simulink model "SimulacaoMassaPonto"  (R2021a)
settings: Solver=VariableStepAuto  StartTime=0.0  StopTime=TVoo  MaxStep=Step  RelTol=1e-3
values from neighbouring files (symbols this model uses):
  g = 9.81    [TesteSimulacaoMP.m]
  Gamma0 = deg2rad(85)    [TesteSimulacaoMP.m]
  Mvazio = 32.3    [TesteSimulacaoMP.m]
  Sref = 0.0196    [TesteSimulacaoMP.m]
  Tq = VProp(end, 1)    [TesteSimulacaoMP.m]
  V0 = 24    [TesteSimulacaoMP.m]
  VCD = [ 0.0 0.3757 ... (first row only)    [TesteSimulacaoMP.m]
  VMass = load('mass.txt')    [TesteSimulacaoMP.m]
  VProp = load('Prop.txt')    [TesteSimulacaoMP.m]
  X0 = deg2rad(45)    [TesteSimulacaoMP.m]
  XEast0 = 0    [TesteSimulacaoMP.m]
  XNorth0 = 0    [TesteSimulacaoMP.m]
  XUp0 = 0    [TesteSimulacaoMP.m]
libraries: simulink x2, simulink_extras x2, aerolibptmass x1, aerolibatmos2 x1
settings Model: Creator=gabriel  LastModifiedBy=gabriel

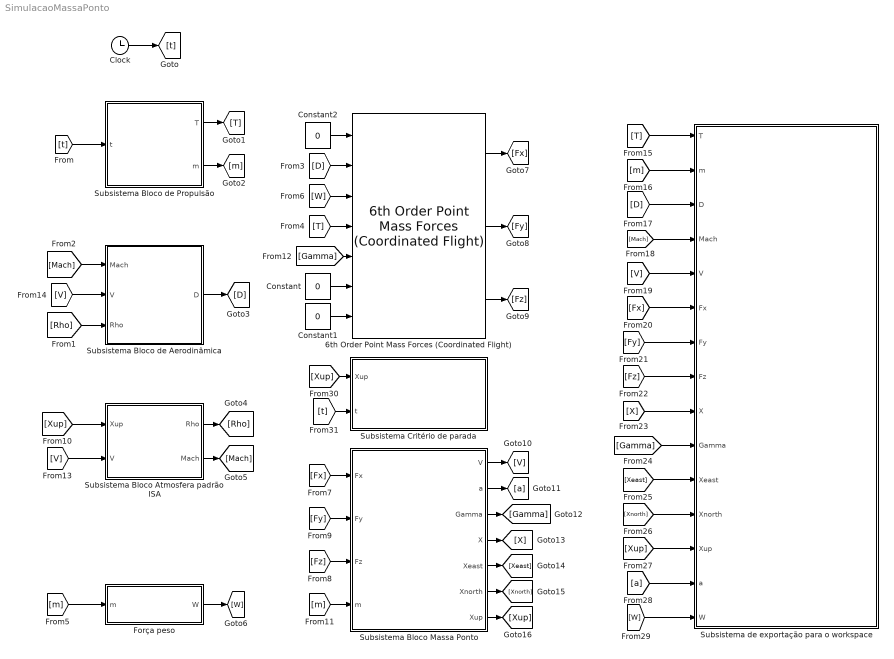
== system SimulacaoMassaPonto ==
  6th Order Point Mass Forces (Coordinated Flight) : aerolibptmass/6th Order Point Mass Forces (Coordinated Flight)
      settings: SourceProductBaseCode=AE
  Clock : Clock
  Constant : Constant  Value=0
  Constant1 : Constant  Value=0
  Constant2 : Constant  Value=0
  Força peso : Subsystem
  Subsistema Bloco Atmosfera padrão ISA : Subsystem
  Subsistema Bloco Massa Ponto : Subsystem
  Subsistema Bloco de Aerodinâmica : Subsystem
  Subsistema Bloco de Propulsão : Subsystem
  Subsistema Critério de parada : Subsystem
  Subsistema de exportação para o workspace : Subsystem
  wires:
  Clock/1 -> [t]
  [t] -> Subsistema Bloco de Propulsão/1(t)
  Subsistema Bloco de Propulsão/1(T) -> [T]
  Subsistema Bloco de Propulsão/2(m) -> [m]
  Subsistema Bloco de Aerodinâmica/1(D) -> [D]
  Subsistema Bloco Atmosfera padrão ISA/1(Rho) -> [Rho]
  [Rho] -> Subsistema Bloco de Aerodinâmica/3(Rho)
  Subsistema Bloco Atmosfera padrão ISA/2(Mach) -> [Mach]
  [Mach] -> Subsistema Bloco de Aerodinâmica/1(Mach)
  [D] -> 6th Order Point Mass Forces (Coordinated Flight)/2
  [T] -> 6th Order Point Mass Forces (Coordinated Flight)/4
  [m] -> Força peso/1(m)
  Força peso/1(W) -> [W]
  [W] -> 6th Order Point Mass Forces (Coordinated Flight)/3
  Constant2/1 -> 6th Order Point Mass Forces (Coordinated Flight)/1
  6th Order Point Mass Forces (Coordinated Flight)/3 -> [Fz]
  6th Order Point Mass Forces (Coordinated Flight)/2 -> [Fy]
  6th Order Point Mass Forces (Coordinated Flight)/1 -> [Fx]
  [Fx] -> Subsistema Bloco Massa Ponto/1(Fx)
  [Fz] -> Subsistema Bloco Massa Ponto/3(Fz)
  [Fy] -> Subsistema Bloco Massa Ponto/2(Fy)
  [m] -> Subsistema Bloco Massa Ponto/4(m)
  Subsistema Bloco Massa Ponto/1(V) -> [V]
  Subsistema Bloco Massa Ponto/2(a) -> [a]
  Subsistema Bloco Massa Ponto/3(Gamma) -> [Gamma]
  [Gamma] -> 6th Order Point Mass Forces (Coordinated Flight)/5
  Constant/1 -> 6th Order Point Mass Forces (Coordinated Flight)/6
  Constant1/1 -> 6th Order Point Mass Forces (Coordinated Flight)/7
  Subsistema Bloco Massa Ponto/4(X) -> [X]
  Subsistema Bloco Massa Ponto/5(Xeast) -> [Xeast]
  Subsistema Bloco Massa Ponto/6(Xnorth) -> [Xnorth]
  Subsistema Bloco Massa Ponto/7(Xup) -> [Xup]
  [Xup] -> Subsistema Bloco Atmosfera padrão ISA/1(Xup)
  [V] -> Subsistema Bloco Atmosfera padrão ISA/2(V)
  [V] -> Subsistema Bloco de Aerodinâmica/2(V)
  [T] -> Subsistema de exportação para o workspace/1(T)
  [m] -> Subsistema de exportação para o workspace/2(m)
  [D] -> Subsistema de exportação para o workspace/3(D)
  [Mach] -> Subsistema de exportação para o workspace/4(Mach)
  [V] -> Subsistema de exportação para o workspace/5(V)
  [Fx] -> Subsistema de exportação para o workspace/6(Fx)
  [Fy] -> Subsistema de exportação para o workspace/7(Fy)
  [Fz] -> Subsistema de exportação para o workspace/8(Fz)
  [X] -> Subsistema de exportação para o workspace/9(X)
  [Gamma] -> Subsistema de exportação para o workspace/10(Gamma)
  [Xeast] -> Subsistema de exportação para o workspace/11(Xeast)
  [Xnorth] -> Subsistema de exportação para o workspace/12(Xnorth)
  [Xup] -> Subsistema de exportação para o workspace/13(Xup)
  [a] -> Subsistema de exportação para o workspace/14(a)
  [W] -> Subsistema de exportação para o workspace/15(W)
  [Xup] -> Subsistema Critério de parada/1(Xup)
  [t] -> Subsistema Critério de parada/2(t)

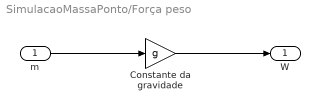
== system SimulacaoMassaPonto/Força peso ==
  m : Inport
  Constante da gravidade : Gain  Gain=g
  W : Outport
  wires:
  m/1 -> Constante da gravidade/1
  Constante da gravidade/1 -> W/1

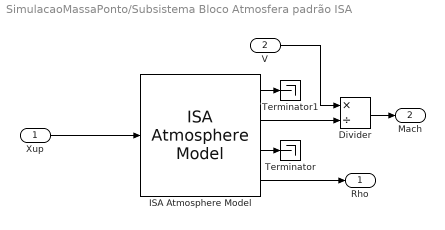
== system SimulacaoMassaPonto/Subsistema Bloco Atmosfera padrão ISA ==
  Xup : Inport
  V : Inport  Port=2
  Divider : Product  Inputs=*/
  ISA Atmosphere Model : aerolibatmos2/ISA Atmosphere Model  custom=off  g=9.80665  gamma=1.4  R=287.0531  L=0.0065  h_trop=11000  h_strat=20000  rho0=1.225  P0=101325  T0=288.15  h0=0
  Terminator : Terminator
  Terminator1 : Terminator
  Rho : Outport
  Mach : Outport  Port=2
  wires:
  Xup/1 -> ISA Atmosphere Model/1
  ISA Atmosphere Model/4 -> Rho/1
  ISA Atmosphere Model/3 -> Terminator/1
  ISA Atmosphere Model/1 -> Terminator1/1
  ISA Atmosphere Model/2 -> Divider/2
  V/1 -> Divider/1
  Divider/1 -> Mach/1

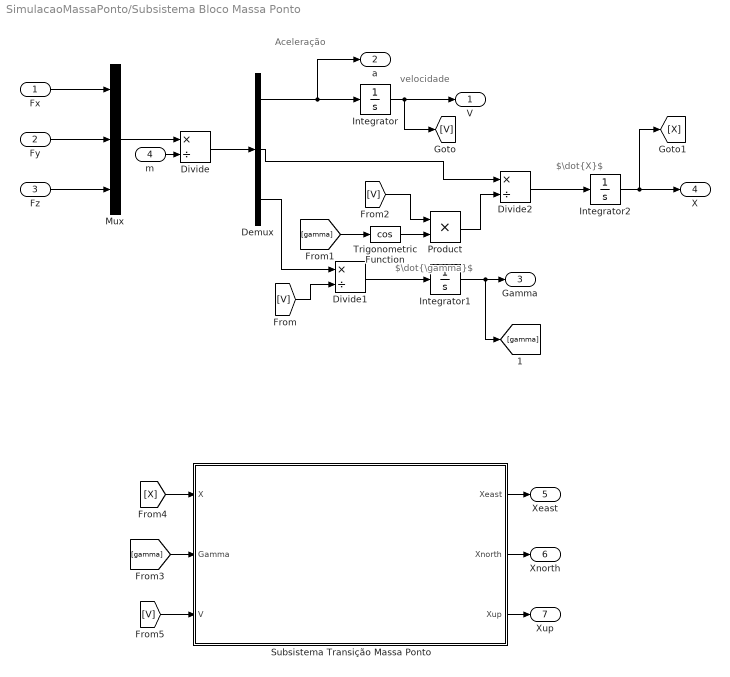
== system SimulacaoMassaPonto/Subsistema Bloco Massa Ponto ==
  note: $\dot{X}$
  note: $\dot{\gamma}$
  note: velocidade
  note: Aceleração
  Fx : Inport
  Fy : Inport  Port=2
  Fz : Inport  Port=3
  m : Inport  Port=4
  Demux : Demux  Outputs=3
  Divide : Product  Inputs=*/
  Divide1 : Product  Inputs=*/
  Divide2 : Product  Inputs=*/
  Integrator : Integrator  InitialCondition=V0
  Integrator1 : Integrator  InitialCondition=Gamma0
  Integrator2 : Integrator  InitialCondition=X0
  Mux : Mux  Inputs=3
  Product : Product
  Subsistema Transição Massa Ponto : Subsystem
  Trigonometric Function : Trigonometry  Operator=cos
  V : Outport
  a : Outport  Port=2
  Gamma : Outport  Port=3
  X : Outport  Port=4
  Xeast : Outport  Port=5
  Xnorth : Outport  Port=6
  Xup : Outport  Port=7
  wires:
  Fy/1 -> Mux/2
  Fx/1 -> Mux/1
  Fz/1 -> Mux/3
  Mux/1 -> Divide/1
  m/1 -> Divide/2
  Divide/1 -> Demux/1
  Demux/1 -> Integrator/1, a/1
  Integrator/1 -> [V], V/1
  Demux/3 -> Divide1/1
  [V] -> Divide1/2
  Divide1/1 -> Integrator1/1
  Integrator1/1 -> [gamma], Gamma/1
  [gamma] -> Trigonometric Function/1
  Trigonometric Function/1 -> Product/2
  [V] -> Product/1
  Demux/2 -> Divide2/1
  Product/1 -> Divide2/2
  Divide2/1 -> Integrator2/1
  Integrator2/1 -> [X], X/1
  [gamma] -> Subsistema Transição Massa Ponto/2(Gamma)
  [X] -> Subsistema Transição Massa Ponto/1(X)
  [V] -> Subsistema Transição Massa Ponto/3(V)
  Subsistema Transição Massa Ponto/3(Xup) -> Xup/1
  Subsistema Transição Massa Ponto/2(Xnorth) -> Xnorth/1
  Subsistema Transição Massa Ponto/1(Xeast) -> Xeast/1

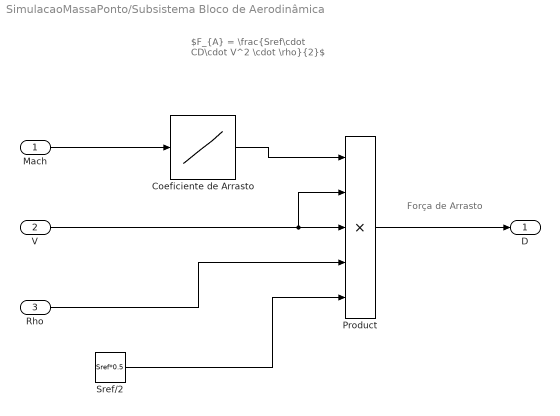
== system SimulacaoMassaPonto/Subsistema Bloco de Aerodinâmica ==
  note: Força de Arrasto
  note: $F_{A} = \frac{Sref\cdot CD\cdot V^2 \cdot \rho}{2}$
  Mach : Inport
  V : Inport  Port=2
  Rho : Inport  Port=3
  Coeficiente de Arrasto : Lookup_n-D  NumberOfTableDimensions=1  BreakpointsForDimension1=VCD(:,1)  Table=VCD(:,2)  ExtrapMethod=Clip  InternalRulePriority=Speed  RndMeth=Simplest  InputSameDT=on
  Product : Product  Inputs=5
  Sref/2 : Constant  Value=Sref*0.5
  D : Outport
  wires:
  Mach/1 -> Coeficiente de Arrasto/1
  Coeficiente de Arrasto/1 -> Product/1
  V/1 -> Product/2, Product/3
  Rho/1 -> Product/4
  Sref/2/1 -> Product/5
  Product/1 -> D/1

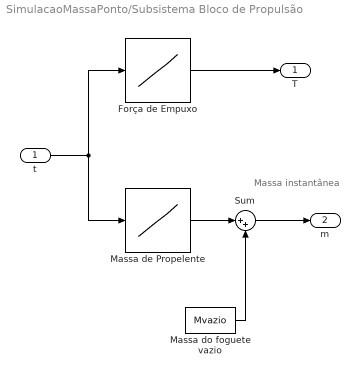
== system SimulacaoMassaPonto/Subsistema Bloco de Propulsão ==
  note: Massa instantânea
  t : Inport
  Força de Empuxo : Lookup_n-D  NumberOfTableDimensions=1  BreakpointsForDimension1=VProp(:,1)  Table=VProp(:,2)  ExtrapMethod=Clip  InternalRulePriority=Speed  RndMeth=Simplest  InputSameDT=on
  Massa de Propelente : Lookup_n-D  NumberOfTableDimensions=1  BreakpointsForDimension1=VMass(:,1)  Table=VMass(:,2)  ExtrapMethod=Clip  InternalRulePriority=Speed  RndMeth=Simplest  InputSameDT=on
  Massa do foguete vazio : Constant  Value=Mvazio
  Sum : Sum  Inputs=|++
  T : Outport
  m : Outport  Port=2
  wires:
  t/1 -> Força de Empuxo/1, Massa de Propelente/1
  Força de Empuxo/1 -> T/1
  Massa de Propelente/1 -> Sum/1
  Massa do foguete vazio/1 -> Sum/2
  Sum/1 -> m/1

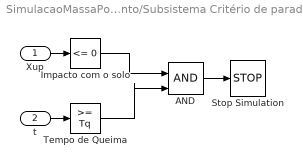
== system SimulacaoMassaPonto/Subsistema Critério de parada ==
  Xup : Inport
  t : Inport  Port=2
  AND : Logic  IconShape=distinctive  AllPortsSameDT=off  OutDataTypeStr=boolean
  Impacto com o solo : simulink/Logic and Bit Operations/Compare To Constant  relop=<=  const=0  OutDataTypeStr=boolean
  Stop Simulation : Stop
  Tempo de Queima : simulink/Logic and Bit Operations/Compare To Constant  relop=>=  const=Tq  OutDataTypeStr=boolean
  wires:
  Xup/1 -> Impacto com o solo/1
  t/1 -> Tempo de Queima/1
  Impacto com o solo/1 -> AND/1
  Tempo de Queima/1 -> AND/2
  AND/1 -> Stop Simulation/1

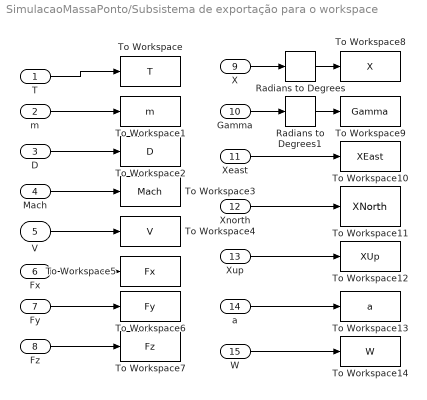
== system SimulacaoMassaPonto/Subsistema de exportação para o workspace ==
  T : Inport
  m : Inport  Port=2
  D : Inport  Port=3
  Mach : Inport  Port=4
  V : Inport  Port=5
  Fx : Inport  Port=6
  Fy : Inport  Port=7
  Fz : Inport  Port=8
  X : Inport  Port=9
  Gamma : Inport  Port=10
  Xeast : Inport  Port=11
  Xnorth : Inport  Port=12
  Xup : Inport  Port=13
  a : Inport  Port=14
  W : Inport  Port=15
  Radians to Degrees : simulink_extras/Transformations/Radians to Degrees
  Radians to Degrees1 : simulink_extras/Transformations/Radians to Degrees
  To Workspace : ToWorkspace  VariableName=T  SampleTime=-1
  To Workspace1 : ToWorkspace  VariableName=m  SampleTime=-1
  To Workspace10 : ToWorkspace  VariableName=XEast  SampleTime=-1
  To Workspace11 : ToWorkspace  VariableName=XNorth  SampleTime=-1
  To Workspace12 : ToWorkspace  VariableName=XUp  SampleTime=-1
  To Workspace13 : ToWorkspace  VariableName=a  SampleTime=-1
  To Workspace14 : ToWorkspace  VariableName=W  SampleTime=-1
  To Workspace2 : ToWorkspace  VariableName=D  SampleTime=-1
  To Workspace3 : ToWorkspace  VariableName=Mach  SampleTime=-1
  To Workspace4 : ToWorkspace  VariableName=V  SampleTime=-1
  To Workspace5 : ToWorkspace  VariableName=Fx  SampleTime=-1
  To Workspace6 : ToWorkspace  VariableName=Fy  SampleTime=-1
  To Workspace7 : ToWorkspace  VariableName=Fz  SampleTime=-1
  To Workspace8 : ToWorkspace  VariableName=X  SampleTime=-1
  To Workspace9 : ToWorkspace  VariableName=Gamma  SampleTime=-1
  wires:
  T/1 -> To Workspace/1
  m/1 -> To Workspace1/1
  D/1 -> To Workspace2/1
  Mach/1 -> To Workspace3/1
  V/1 -> To Workspace4/1
  Fx/1 -> To Workspace5/1
  Fy/1 -> To Workspace6/1
  Fz/1 -> To Workspace7/1
  X/1 -> Radians to Degrees/1
  Gamma/1 -> Radians to Degrees1/1
  Xeast/1 -> To Workspace10/1
  Radians to Degrees/1 -> To Workspace8/1
  Radians to Degrees1/1 -> To Workspace9/1
  Xnorth/1 -> To Workspace11/1
  Xup/1 -> To Workspace12/1
  a/1 -> To Workspace13/1
  W/1 -> To Workspace14/1

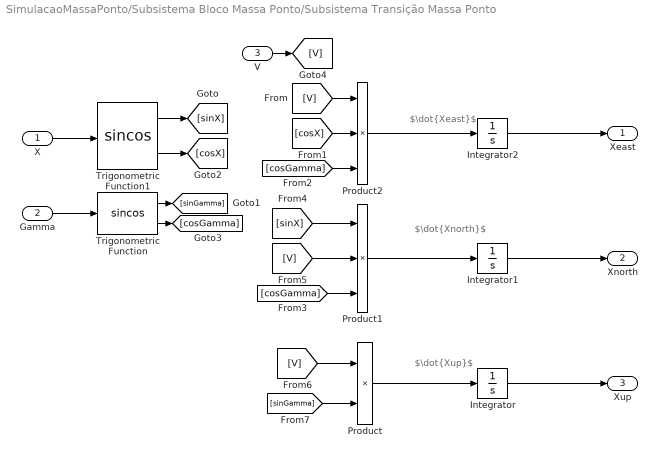
== system SimulacaoMassaPonto/Subsistema Bloco Massa Ponto/Subsistema Transição Massa Ponto ==
  note: $\dot{Xeast}$
  note: $\dot{Xnorth}$
  note: $\dot{Xup}$
  X : Inport
  Gamma : Inport  Port=2
  V : Inport  Port=3
  Integrator : Integrator  InitialCondition=XUp0
  Integrator1 : Integrator  InitialCondition=XNorth0
  Integrator2 : Integrator  InitialCondition=XEast0
  Product : Product
  Product1 : Product  Inputs=3
  Product2 : Product  Inputs=3
  Trigonometric Function : Trigonometry  Operator=sincos
  Trigonometric Function1 : Trigonometry  Operator=sincos
  Xeast : Outport
  Xnorth : Outport  Port=2
  Xup : Outport  Port=3
  wires:
  X/1 -> Trigonometric Function1/1
  Gamma/1 -> Trigonometric Function/1
  Trigonometric Function/1 -> [sinGamma]
  Trigonometric Function/2 -> [cosGamma]
  Trigonometric Function1/1 -> [sinX]
  Trigonometric Function1/2 -> [cosX]
  V/1 -> [V]
  Product/1 -> Integrator/1
  Integrator/1 -> Xup/1
  Product2/1 -> Integrator2/1
  Integrator2/1 -> Xeast/1
  Integrator1/1 -> Xnorth/1
  Product1/1 -> Integrator1/1
  [V] -> Product2/1
  [cosX] -> Product2/2
  [cosGamma] -> Product2/3
  [V] -> Product1/2
  [sinX] -> Product1/1
  [cosGamma] -> Product1/3
  [V] -> Product/1
  [sinGamma] -> Product/2
